simulink model "vib_sim1"  (Simulink 7.9)
settings: Solver=ode4  StartTime=0.0  StopTime=t  FixedStep=tt  RelTol=1e-3
values from neighbouring files (symbols this model uses):
  c = 20.7    [Mycode.m]    (also in vib2.m = 10)
  f = 500    [Mycode.m]    (also in vib2.m = 400)
  k = 1140    [Mycode.m]    (also in vib2.m = 10000)
  m = 5.7    [Mycode.m]    (also in vib2.m = 2)
  tt = 0.01    [Mycode.m]    (also in vib2.m)
  w = 0    [Mycode.m]    (also in vib2.m)
settings Model: Creator=Zahid  LastModifiedBy=User

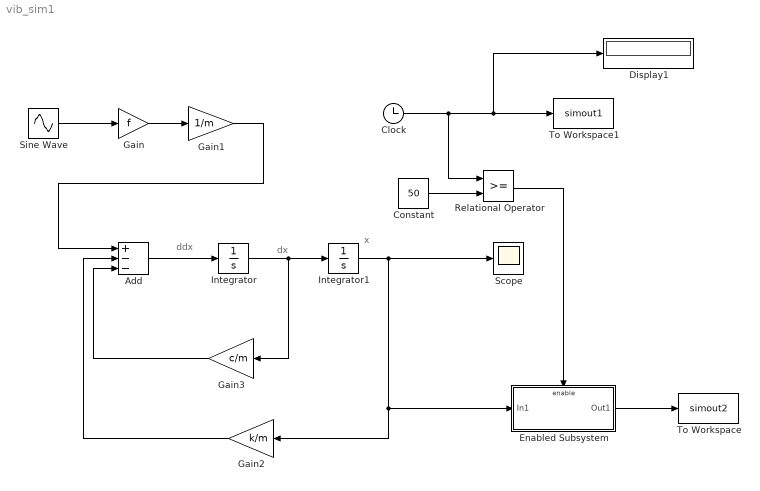
== system vib_sim1 ==
  note: ddx
  note: dx
  note: x
  Add : Sum  Inputs=+--
  Clock : Clock
  Constant : Constant  Value=50
  Display1 : Display
  Enabled Subsystem : Subsystem  TreatAsAtomicUnit=on
  Gain : Gain  Gain=f
  Gain1 : Gain  Gain=1/m
  Gain2 : Gain  Gain=k/m
  Gain3 : Gain  Gain=c/m
  Integrator : Integrator
  Integrator1 : Integrator
  Relational Operator : RelationalOperator  OutDataTypeStr=boolean
  Scope : Scope
      settings: SampleInput=on  SampleTime=tt
  Sine Wave : Sin  Frequency=w  SampleTime=tt
  To Workspace : ToWorkspace  VariableName=simout2  SampleTime=-1
  To Workspace1 : ToWorkspace  VariableName=simout1  SampleTime=tt
  wires:
  Sine Wave/1 -> Gain/1
  Gain/1 -> Gain1/1
  Gain1/1 -> Add/1
  Add/1 -> Integrator/1
  Integrator/1 -> Integrator1/1, Gain3/1
  Integrator1/1 -> Scope/1, Gain2/1, Enabled Subsystem/1(In1)
  Gain2/1 -> Add/2
  Gain3/1 -> Add/3
  Clock/1 -> To Workspace1/1, Display1/1, Relational Operator/1
  Enabled Subsystem/1(Out1) -> To Workspace/1
  Constant/1 -> Relational Operator/2
  Relational Operator/1 -> Enabled Subsystem/Enable

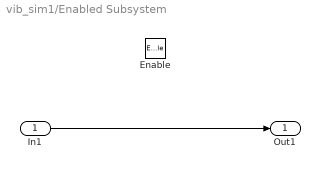
== system vib_sim1/Enabled Subsystem ==
  In1 : Inport
  Enable : EnablePort
  Out1 : Outport
  wires:
  In1/1 -> Out1/1
